simulink model "stage2simulink-viral"  (R2018b)
settings: Solver=VariableStepAuto  StartTime=0.0  StopTime=50  RelTol=1e-3
values from neighbouring files (symbols this model uses):
  C = Q/(1-Q*g1)    [part2-viral.m]    (also in part2_Nathan.m; qdesign-viral.m)
  delay_ss1 = 0.7    [part2-viral.m]    (also in part2.m; part2_Nathan.m; qdesign-viral.m)
  g1 = tf(ss1_num,ss1_den)    [part2-viral.m]    (also in part2.m; part2_Nathan.m; qdesign-viral.m)
  lower_lim = -2.5    [part2-viral.m]    (also in part2.m; part2_Nathan.m; qdesign-viral.m)
  ss1_den = [1.8 4.5 1]    [part2-viral.m]    (also in part2.m; part2_Nathan.m; qdesign-viral.m)
  ss1_num = 0.1    [part2-viral.m]    (also in part2.m; part2_Nathan.m; qdesign-viral.m)
  upper_lim = 2.5    [part2-viral.m]    (also in part2.m; part2_Nathan.m; qdesign-viral.m)
libraries: cstblocks x14, dspinverses x1
settings Model: Creator=viral  LastModifiedBy=viral

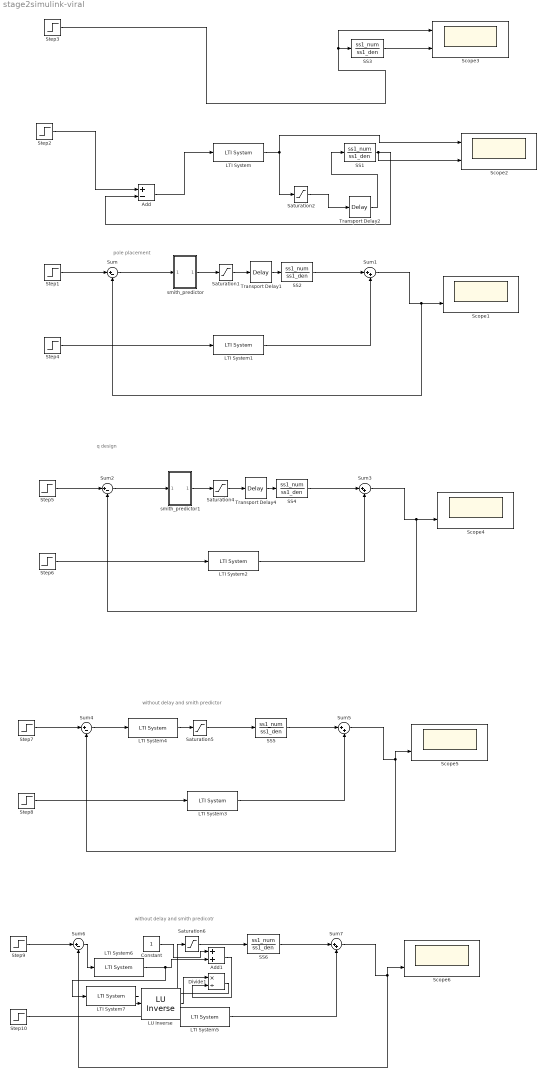
== system stage2simulink-viral ==
  note: pole placement
  note: q design
  note: without delay and smith predictor
  note: without delay and smith predicotr
  " LU Inverse" : dspinverses/ LU Inverse
      settings: SourceProductName=DSP System Toolbox
  Add : Sum  Inputs=+-
  Add1 : Sum
  Constant : Constant
  Divide1 : Product  Inputs=*/
  LTI System : cstblocks/LTI System  sys=pid  IC=[]
  LTI System{1..3,5} (4 alike) : cstblocks/LTI System  sys=g2  IC=[]
  LTI System4 : cstblocks/LTI System  sys=C  IC=[]
  LTI System6 : cstblocks/LTI System  sys=F  IC=[]
  LTI System7 : cstblocks/LTI System  sys=g1  IC=[]
  SS{1..6} (6 alike) : TransferFcn  Numerator=ss1_num  Denominator=ss1_den
  Saturation{1..2,4..6} (5 alike) : Saturate  UpperLimit=upper_lim  LowerLimit=lower_lim
  Scope{1..6} (6 alike) : Scope  NumInputPorts=2
  Step{1..2,5,7,9} (5 alike) : Step  Time=5  SampleTime=0
  Step{4,6,8,10} (4 alike) : Step  Time=25  After=0.1  SampleTime=0
  Step3 : Step  Time=5  After=2.5  SampleTime=0
  Sum{,2,4,6} (4 alike) : Sum  Inputs=|+-
  Sum{1,3,5,7} (4 alike) : Sum  Inputs=|++
  Transport Delay1 : TransportDelay  DelayTime=delay_ss1
  Transport Delay2 : TransportDelay  DelayTime=delay_ss1
  Transport Delay4 : TransportDelay  DelayTime=delay_ss1
  smith_predictor : Subsystem
  smith_predictor1 : Subsystem
  wires:
  Transport Delay1/1 -> SS2/1
  SS1/1 -> Add/2, Scope2/2
  Transport Delay2/1 -> SS1/1
  Step3/1 -> Scope3/1, SS3/1
  SS3/1 -> Scope3/2
  Step1/1 -> Sum/1
  Step2/1 -> Add/1
  Add/1 -> LTI System/1
  Sum/1 -> smith_predictor/1(In1)
  smith_predictor/1(Out1) -> Saturation1/1
  Saturation1/1 -> Transport Delay1/1
  LTI System/1 -> Saturation2/1, Scope2/1
  Saturation2/1 -> Transport Delay2/1
  Step4/1 -> LTI System1/1
  Sum1/1 -> Sum/2, Scope1/2
  LTI System1/1 -> Sum1/2
  SS2/1 -> Sum1/1
  Saturation4/1 -> Transport Delay4/1
  Step5/1 -> Sum2/1
  Sum3/1 -> Sum2/2, Scope4/2
  Step6/1 -> LTI System2/1
  LTI System2/1 -> Sum3/2
  Transport Delay4/1 -> SS4/1
  Sum2/1 -> smith_predictor1/1(In1)
  smith_predictor1/1(Out1) -> Saturation4/1
  SS4/1 -> Sum3/1
  Step8/1 -> LTI System3/1
  SS5/1 -> Sum5/1
  Step7/1 -> Sum4/1
  Sum5/1 -> Sum4/2, Scope5/2
  LTI System3/1 -> Sum5/2
  Saturation5/1 -> SS5/1
  Sum4/1 -> LTI System4/1
  LTI System4/1 -> Saturation5/1
  Step9/1 -> Sum6/1
  Sum6/1 -> LTI System6/1
  Step10/1 -> LTI System5/1
  SS6/1 -> Sum7/1
  Saturation6/1 -> SS6/1
  Sum7/1 -> Sum6/2, Scope6/2
  LTI System5/1 -> Sum7/2
  Divide1/1 -> Saturation6/1
  LTI System6/1 -> LTI System7/1, Add1/2
  Constant/1 -> Add1/1
  Add1/1 -> Divide1/2
  LTI System7/1 -> " LU Inverse"/1
  " LU Inverse"/1 -> Divide1/1

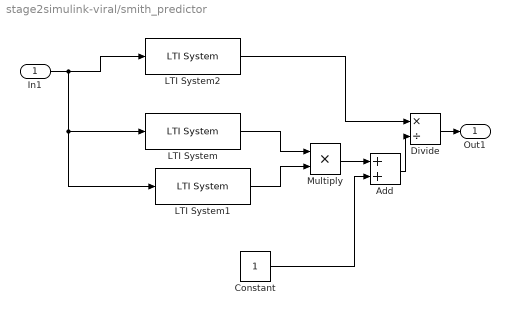
== system stage2simulink-viral/smith_predictor ==
  In1 : Inport
  Add : Sum
  Constant : Constant
  Divide : Product  Inputs=*/
  LTI System : cstblocks/LTI System  sys=c1g1  IC=[]
  LTI System1 : cstblocks/LTI System  sys=temp  IC=[]
  LTI System2 : cstblocks/LTI System  sys=c1  IC=[]
  Multiply : Product
  Out1 : Outport
  wires:
  LTI System1/1 -> Multiply/2
  LTI System2/1 -> Divide/1
  LTI System/1 -> Multiply/1
  Divide/1 -> Out1/1
  In1/1 -> LTI System1/1, LTI System/1, LTI System2/1
  Multiply/1 -> Add/1
  Constant/1 -> Add/2
  Add/1 -> Divide/2

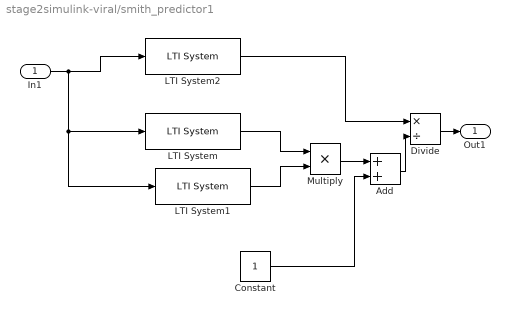
== system stage2simulink-viral/smith_predictor1 ==
  In1 : Inport
  Add : Sum
  Constant : Constant
  Divide : Product  Inputs=*/
  LTI System : cstblocks/LTI System  sys=C*g1  IC=[]
  LTI System1 : cstblocks/LTI System  sys=temp  IC=[]
  LTI System2 : cstblocks/LTI System  sys=C  IC=[]
  Multiply : Product
  Out1 : Outport
  wires:
  LTI System1/1 -> Multiply/2
  LTI System2/1 -> Divide/1
  LTI System/1 -> Multiply/1
  Divide/1 -> Out1/1
  In1/1 -> LTI System1/1, LTI System/1, LTI System2/1
  Multiply/1 -> Add/1
  Constant/1 -> Add/2
  Add/1 -> Divide/2
